simulink model "Arti_DeltaSM_Control_Fricc"  (R2014a)
settings: Solver=ode15s  StartTime=0.0  StopTime=TSimulacion  FixedStep=0.0005  RelTol=1e-3
InitFcn:
  | Px1=  [  -70,  -70,   140,  140  ];
  | Pz1=  [-300, -160,- 160, -300];
  | Py1=  [     0,      0,     0,      0];
  | Fs2=0.01;
  | Fc2=0.01;
  | load('C:\Users\Sebastian\Desktop\T_SM\Modelado_Motores\Modelo Completo\WorkSpace-Resultados\EstimacionconFriccionCnts.mat')
  | 
  | 
  | % Calculo de valores intermedios y tiempo inicial
  | Px= tercios(Px1);
  | Pz= tercios(Pz1);
  | Py= tercios(Py1);
  | Tiempo=(1:length(Px)-1)*0+0.1;
  | 
  | %calculo de angulos
  | [Th1(1),Th2(1), Th3(1)] =ArtiCinInv(Px(1), Py(1), Pz(1),0,0, 0);
  | for i=2:length(Px)
  |      [Th1(i),Th2(i), Th3(i)] =ArtiCinInv(Px(i), Py(i), Pz(i),Th1(i-1),Th2(i-1), Th3(i-1));
  | end
  | 
  | 
  | 
  | %syncronizar
  | Tiempo=SyncronizarTiempos(Th1,Tiempo);
  | Tiempo=SyncronizarTiempos(Th2,Tiempo);
  | Tiempo=SyncronizarTiempos(Th3,Tiempo);
  | 
  | A1=CalculoPolinomios(Th1,Tiempo);
  | A2=CalculoPolinomios(Th2,Tiempo);
  | A3=CalculoPolinomios(Th3,Tiempo);
  | 
  | TiempoAcu=[0,cumsum(Tiempo)];
  | TSimulacion=floor((TiempoAcu(end)*100))/100
undefined symbols (not defined in the file): G, Ilimit, TLimit, X, Y, Z
libraries: sm_lib x238, Fricciones x15, nesl_utility x10, simulink x3
(part 6 of 6)

== system Arti_DeltaSM_Control_Fricc/DeltaSM/BaseMovil/acopleBaseMovilAntebrazo_3_RIGID/ball_Uniball_1_RIGID ==
  ReferenceFrame : sm_lib/Frames and Transforms/Reference Frame  BlockFunction=simmechanics.library.frames_transforms.reference_frame
  Solid : sm_lib/Body Elements/Solid  InertiaType=Custom  Mass=0.0055458151739754217  MassUnits=kg  CenterOfMass=[-2.6002689251073309e-05 0 0]  CenterOfMassUnits=mm  MomentsOfInertia=[0.091219033457233048 0.091225744336999384 0.12400458181757036]  MomentsOfInertiaUnits=kg*mm^2  ProductsOfInertia=[0 0 0]  ProductsOfInertiaUnits=kg*mm^2  DensityBased=on  Density=1000  DensityUnits=kg/(m^3)  GraphicType=FromGeometry  MarkerShape=Sphere  MarkerSize=10  MarkerSizeUnits=m  GraphicVisPropType=SimpleVisualProperties  GraphicDiffuseColor=[0.89803921568627454 0.89803921568627454 0.89803921568627454]  GraphicSpecularColor=[0.5 0.5 0.5 1.0]  GraphicAmbientColor=[0.15 0.15 0.15 1.0]  GraphicEmissiveColor=[0.0 0.0 0.0 1.0]  GraphicShininess=75  GraphicOpacity=1  GeometryShape=FromFile  RectangleSize=[1 1]  RectangleSizeUnits=m  BrickDimensions=[1 1 1]  BrickDimensionUnits=m  CylinderRadius=1  CylinderRadiusUnits=m  CylinderLength=1  CylinderLengthUnits=m  SphereRadius=1  SphereRadiusUnits=m  EllipsoidRadii=[1 1 1]  EllipsoidRadiiUnits=m  ExtrusionCrossSection=[1 1; -1 1; -1 -1; 1 -1]  ExtrusionCrossSectionUnits=m  ExtrusionLength=1  ExtrusionLengthUnits=m  PolygonNumSides=3  PolygonOuterRadius=1  PolygonOuterRadiusUnits=m  ExtGeomFileType=STL  ExtGeomFileName=ball_Uniball_?? ?????????_sldprt.STL  ExtGeomFileUnits=mm  RevolutionCrossSection=[1 1; 1 -1; 2 -1; 2 1]  RevolutionCrossSectionUnits=m  RevolutionExtent=Full  RevolutionAngle=180  RevolutionAngleUnits=deg  BlockFunction=simmechanics.library.body_elements.solid
  F : PMIOPort  Port=1  Side=Left
  connections:
  ReferenceFrame/RConn1 -- Solid/RConn1 -- F/RConn1

== system Arti_DeltaSM_Control_Fricc/DeltaSM/BaseMovil/acopleBaseMovilAntebrazo_3_RIGID/ball_Uniball_2_RIGID ==
  ReferenceFrame : sm_lib/Frames and Transforms/Reference Frame  BlockFunction=simmechanics.library.frames_transforms.reference_frame
  Solid : sm_lib/Body Elements/Solid  InertiaType=Custom  Mass=0.0055458151739754217  MassUnits=kg  CenterOfMass=[-2.6002689251073309e-05 0 0]  CenterOfMassUnits=mm  MomentsOfInertia=[0.091219033457233048 0.091225744336999384 0.12400458181757036]  MomentsOfInertiaUnits=kg*mm^2  ProductsOfInertia=[0 0 0]  ProductsOfInertiaUnits=kg*mm^2  DensityBased=on  Density=1000  DensityUnits=kg/(m^3)  GraphicType=FromGeometry  MarkerShape=Sphere  MarkerSize=10  MarkerSizeUnits=m  GraphicVisPropType=SimpleVisualProperties  GraphicDiffuseColor=[0.89803921568627454 0.89803921568627454 0.89803921568627454]  GraphicSpecularColor=[0.5 0.5 0.5 1.0]  GraphicAmbientColor=[0.15 0.15 0.15 1.0]  GraphicEmissiveColor=[0.0 0.0 0.0 1.0]  GraphicShininess=75  GraphicOpacity=1  GeometryShape=FromFile  RectangleSize=[1 1]  RectangleSizeUnits=m  BrickDimensions=[1 1 1]  BrickDimensionUnits=m  CylinderRadius=1  CylinderRadiusUnits=m  CylinderLength=1  CylinderLengthUnits=m  SphereRadius=1  SphereRadiusUnits=m  EllipsoidRadii=[1 1 1]  EllipsoidRadiiUnits=m  ExtrusionCrossSection=[1 1; -1 1; -1 -1; 1 -1]  ExtrusionCrossSectionUnits=m  ExtrusionLength=1  ExtrusionLengthUnits=m  PolygonNumSides=3  PolygonOuterRadius=1  PolygonOuterRadiusUnits=m  ExtGeomFileType=STL  ExtGeomFileName=ball_Uniball_?? ?????????_sldprt.STL  ExtGeomFileUnits=mm  RevolutionCrossSection=[1 1; 1 -1; 2 -1; 2 1]  RevolutionCrossSectionUnits=m  RevolutionExtent=Full  RevolutionAngle=180  RevolutionAngleUnits=deg  BlockFunction=simmechanics.library.body_elements.solid
  F : PMIOPort  Port=1  Side=Left
  connections:
  ReferenceFrame/RConn1 -- Solid/RConn1 -- F/RConn1
